simulink model "dcMotorSim"  (R2021b)
settings: Solver=VariableStepAuto  StartTime=0.0  StopTime=10  RelTol=1e-3
values from neighbouring files (symbols this model uses):
  J = 0.181    [dcMotorPar.m]
  kb = 36.9e-3    (= 0.0369)    [dcMotorPar.m]
  kf = 0.1    [dcMotorPar.m]
  km = 20    [dcMotorPar.m]
  L = 0.463e-3    (= 0.000463)    [dcMotorPar.m]
  R = 0.608    [dcMotorPar.m]
settings Model: Creator=chsl  LastModifiedBy=Thomas Therkelsen
settings SolverCC: AlgebraicLoopSolver=TrustRegion
settings DataIOCC: ReturnWorkspaceOutputs=off
settings DebuggingCC: SFMachineParentedDataDiag=warning  ArithmeticOperatorsInVariantConditions=warning
settings SFSimCC: SimUseLocalCustomCode=off  CustomCodeUndefinedFunction=UseInterfaceOnly
settings RTWCC: RTWUseLocalCustomCode=off

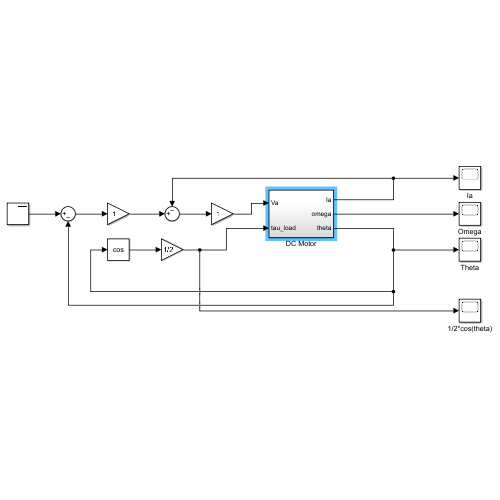
[thumbnail: Simulink's stored preview of the top-level diagram]
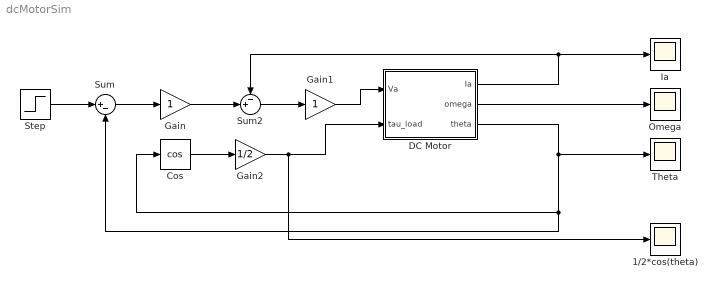
== system dcMotorSim ==
  1/2*cos(theta) : Scope
  Cos : Trigonometry  Operator=cos
  DC Motor : Subsystem
  Gain : Gain
  Gain1 : Gain
  Gain2 : Gain  Gain=1/2
  Ia : Scope
  Omega : Scope
  Step : Step  SampleTime=0
  Sum : Sum  Inputs=|+-
  Sum2 : Sum  Inputs=-+|
  Theta : Scope
  wires:
  DC Motor/3(theta) -> Cos/1, Sum/2, Theta/1
  DC Motor/1(Ia) -> Sum2/1, Ia/1
  DC Motor/2(omega) -> Omega/1
  Step/1 -> Sum/1
  Sum/1 -> Gain/1
  Sum2/1 -> Gain1/1
  Gain1/1 -> DC Motor/1(Va)
  Gain/1 -> Sum2/2
  Cos/1 -> Gain2/1
  Gain2/1 -> 1/2*cos(theta)/1, DC Motor/2(tau_load)

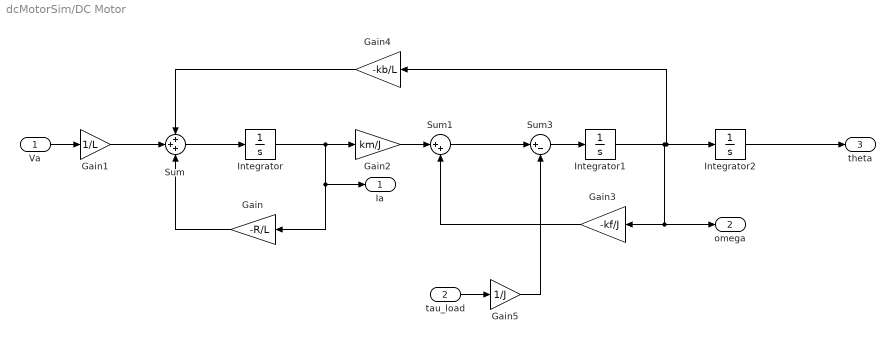
== system dcMotorSim/DC Motor ==
  Va : Inport
  tau_load : Inport  Port=2
  Gain : Gain  Gain=-R/L
  Gain1 : Gain  Gain=1/L
  Gain2 : Gain  Gain=km/J
  Gain3 : Gain  Gain=-kf/J
  Gain4 : Gain  Gain=-kb/L
  Gain5 : Gain  Gain=1/J
  Integrator : Integrator
  Integrator1 : Integrator
  Integrator2 : Integrator
  Sum : Sum  Inputs=+++
  Sum1 : Sum  Inputs=|++
  Sum3 : Sum  Inputs=|+-
  Ia : Outport  VectorParamsAs1DForOutWhenUnconnected=off
  omega : Outport  Port=2  VectorParamsAs1DForOutWhenUnconnected=off
  theta : Outport  Port=3  VectorParamsAs1DForOutWhenUnconnected=off
  wires:
  Gain2/1 -> Sum1/1
  Integrator/1 -> Ia/1, Gain/1, Gain2/1
  Sum/1 -> Integrator/1
  Va/1 -> Gain1/1
  Gain1/1 -> Sum/2
  Gain3/1 -> Sum1/2
  Gain4/1 -> Sum/1
  Sum1/1 -> Sum3/1
  Gain/1 -> Sum/3
  Integrator2/1 -> theta/1
  tau_load/1 -> Gain5/1
  Sum3/1 -> Integrator1/1
  Integrator1/1 -> Gain3/1, omega/1, Gain4/1, Integrator2/1
  Gain5/1 -> Sum3/2
